simulink model "CruiseControl_Headway"  (R2022a)
settings: Solver=ode1  StartTime=0.0  StopTime=600.0  FixedStep=0.1  RelTol=1e-3  EnableMultiTasking=on
values from neighbouring files (symbols this model uses):
  J = lqr(A,B,Q,R)    [LQR_script.m]
settings Model: Creator=burl  LastModifiedBy=prajw
settings SolverCC: AlgebraicLoopSolver=TrustRegion
settings DataIOCC: ReturnWorkspaceOutputs=off
settings OptimizationCC: LifeSpan=inf
settings DebuggingCC: UnconnectedInputMsg=warning  UnconnectedOutputMsg=warning  UnconnectedLineMsg=warning  SFUnexpectedBacktrackingDiag=warning  SFNoUnconditionalDefaultTransitionDiag=warning  SFExecutionAtInitializationDiag=none  SFMachineParentedDataDiag=warning  ArithmeticOperatorsInVariantConditions=warning
settings SFSimCC: SimUseLocalCustomCode=off  CustomCodeUndefinedFunction=UseInterfaceOnly
settings RTWCC: RTWUseLocalCustomCode=off
settings CodeAppCC: StateflowObjectComments=on
settings GRTTargetCC: TargetLangStandard=C89/C90 (ANSI)
settings ConfigComp: CovMetricSettings=dw  CovSaveCumulativeToWorkspaceVar=on  CovSaveSingleToWorkspaceVar=on  CovExternalEMLEnable=off

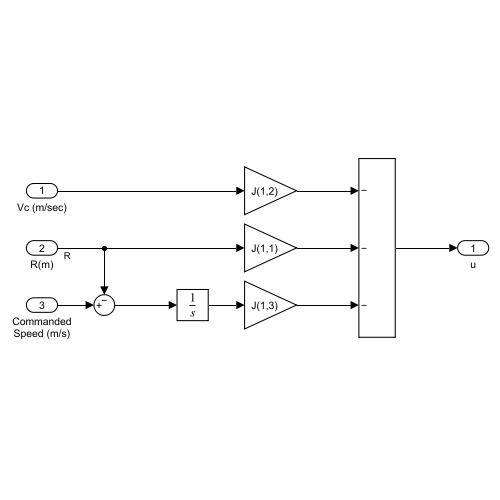
[thumbnail: Simulink's stored preview of the top-level diagram]
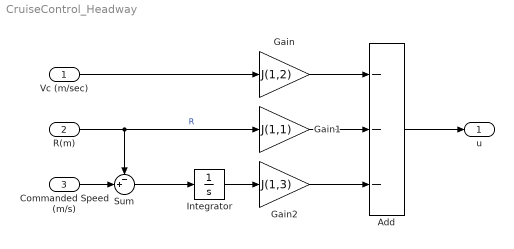
== system CruiseControl_Headway ==
  Vc (m/sec) : Inport
  R(m) : Inport  Port=2
  Commanded Speed (m/s) : Inport  Port=3
  Add : Sum  Inputs=---
  Gain : Gain  Gain=J(1,2)
  Gain1 : Gain  Gain=J(1,1)
  Gain2 : Gain  Gain=J(1,3)
  Integrator : Integrator
  Sum : Sum  Inputs=-+|
  u : Outport  VectorParamsAs1DForOutWhenUnconnected=off
  wires:
  Add/1 -> u/1
  Vc (m/sec)/1 -> Gain/1
  Gain/1 -> Add/1
  R(m)/1 -> Sum/1, Gain1/1  "R"
  Gain1/1 -> Add/2
  Commanded Speed (m/s)/1 -> Sum/2
  Sum/1 -> Integrator/1
  Integrator/1 -> Gain2/1
  Gain2/1 -> Add/3
